simulink model "identificacionPrametros"  (R2014b)
settings: Solver=ode45  StartTime=0.0  StopTime=10.0  RelTol=1e-3
undefined symbols (not defined in the file): a, b
libraries: simulink x1
settings Model: Creator=roberto  LastModifiedBy=roberto

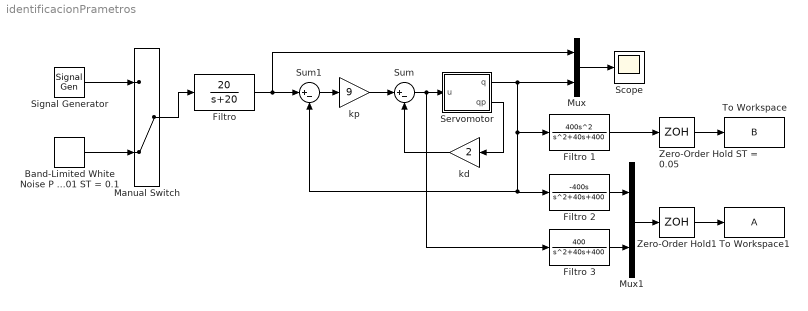
== system identificacionPrametros ==
  Band-Limited White Noise P = 0.01 ST = 0.1 : simulink/Sources/Band-Limited White Noise  Cov=[0.01]  Ts=0.1  seed=[23341]
  Filtro : TransferFcn  Numerator=[20]  Denominator=[1 20]
  Filtro 1 : TransferFcn  Numerator=[400 0 0]  Denominator=[1 40 400]
  Filtro 2 : TransferFcn  Numerator=[-400 0 ]  Denominator=[1 40 400]
  Filtro 3 : TransferFcn  Numerator=[400]  Denominator=[1 40 400]
  Manual Switch : ManualSwitch  CurrentSetting=0
  Mux : Mux  Inputs=2
  Mux1 : Mux  Inputs=2
  Scope : Scope
  Servomotor : Subsystem
  Signal Generator : SignalGenerator  WaveForm=square  Amplitude=0.1  Frequency=0.25
  Sum : Sum  Inputs=|+-
  Sum1 : Sum  Inputs=|+-
  To Workspace : ToWorkspace  VariableName=B  SaveFormat=Timeseries  SampleTime=-1
  To Workspace1 : ToWorkspace  VariableName=A  SaveFormat=Timeseries  SampleTime=-1
  Zero-Order Hold ST = 0.05 : ZeroOrderHold  SampleTime=0.05
  Zero-Order Hold1 : ZeroOrderHold  SampleTime=0.05
  kd : Gain  Gain=2
  kp : Gain  Gain=9
  wires:
  Mux/1 -> Scope/1
  Sum/1 -> Filtro 3/1, Servomotor/1(u)
  Servomotor/2(qp) -> kd/1
  kd/1 -> Sum/2
  kp/1 -> Sum/1
  Sum1/1 -> kp/1
  Servomotor/1(q) -> Mux/2, Filtro 1/1, Filtro 2/1, Sum1/2
  Filtro/1 -> Mux/1, Sum1/1
  Manual Switch/1 -> Filtro/1
  Signal Generator/1 -> Manual Switch/1
  Band-Limited White Noise P = 0.01 ST = 0.1/1 -> Manual Switch/2
  Filtro 2/1 -> Mux1/1
  Filtro 3/1 -> Mux1/2
  Filtro 1/1 -> Zero-Order Hold ST = 0.05/1
  Mux1/1 -> Zero-Order Hold1/1
  Zero-Order Hold ST = 0.05/1 -> To Workspace/1
  Zero-Order Hold1/1 -> To Workspace1/1

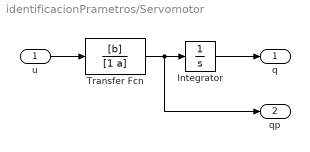
== system identificacionPrametros/Servomotor ==
  u : Inport
  Integrator : Integrator
  Transfer Fcn : TransferFcn  Numerator=[b]  Denominator=[1 a]
  q : Outport
  qp : Outport  Port=2
  wires:
  Integrator/1 -> q/1
  u/1 -> Transfer Fcn/1
  Transfer Fcn/1 -> qp/1, Integrator/1
